simulink model "STATEFLOW"  (R2024b)
settings: Solver=FixedStepAuto  StartTime=0.0  StopTime=10.0  RelTol=1e-3  EnableMultiTasking=on
settings Model: DataDictionary=Master_Dictionary.sldd  EnableAccessToBaseWorkspace=off  Creator=torni  LastModifiedBy=Will
settings OptimizationCC: DefaultParameterBehavior=Inlined  EnhancedBackFolding=on  PassReuseOutputArgsAs=Individual arguments  ZeroExternalMemoryAtStartup=off  ZeroInternalMemoryAtStartup=off  MaxStackSize=8192  OptimizeBlockOrder=speed  DifferentSizesBufferReuse=on  OptimizationCustomize=off  EfficientTunableParamExpr=on
settings DebuggingCC: ParameterTunabilityLossMsg=error
settings HardwareCC: ProdBitPerPointer=32  ProdBitPerSizeT=32  ProdBitPerPtrDiffT=32  ProdLargestAtomicInteger=Long  ProdLargestAtomicFloat=Double  ProdWordSize=32  ProdLongLongMode=on  ProdHWDeviceType=ARM Compatible->ARM Cortex-M
settings SFSimCC: MATLABDynamicMemAlloc=off
settings RTWCC: Description=Embedded Coder  SystemTargetFile=ert.tlc  HardwareBoard=STM32H7xx Based (Single-core)  TemplateMakefile=ert_default_tmf  Toolchain=GNU Tools for ARM Embedded Processors
settings CodeAppCC: ForceParamTrailComments=on  IgnoreCustomStorageClasses=off  OperatorAnnotations=on  SimulinkDataObjDesc=on  SFDataObjDesc=on  InsertBlockDesc=on
settings ERTTargetCC: TargetLangStandard=C99 (ISO)  CodeReplacementLibrary=ARM Cortex-M  ExtModeTransport=3  ExtModeStaticAlloc=on  ExtModeStaticAllocSize=2048  ExtModeMexFile=ext_xcp  ExtModeIntrfLevel=Level2 - Open

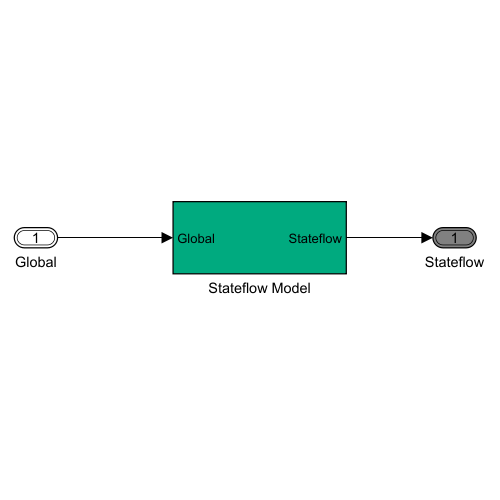
[thumbnail: Simulink's stored preview of the top-level diagram]
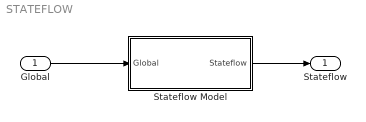
== system STATEFLOW ==
  "Global " : Inport  OutDataTypeStr=Bus: Global
  Stateflow Model : Subsystem
  Stateflow : Outport  OutDataTypeStr=Bus: Stateflow  VectorParamsAs1DForOutWhenUnconnected=off
  wires:
  "Global "/1 -> Stateflow Model/1(Global)
  Stateflow Model/1(Stateflow) -> Stateflow/1

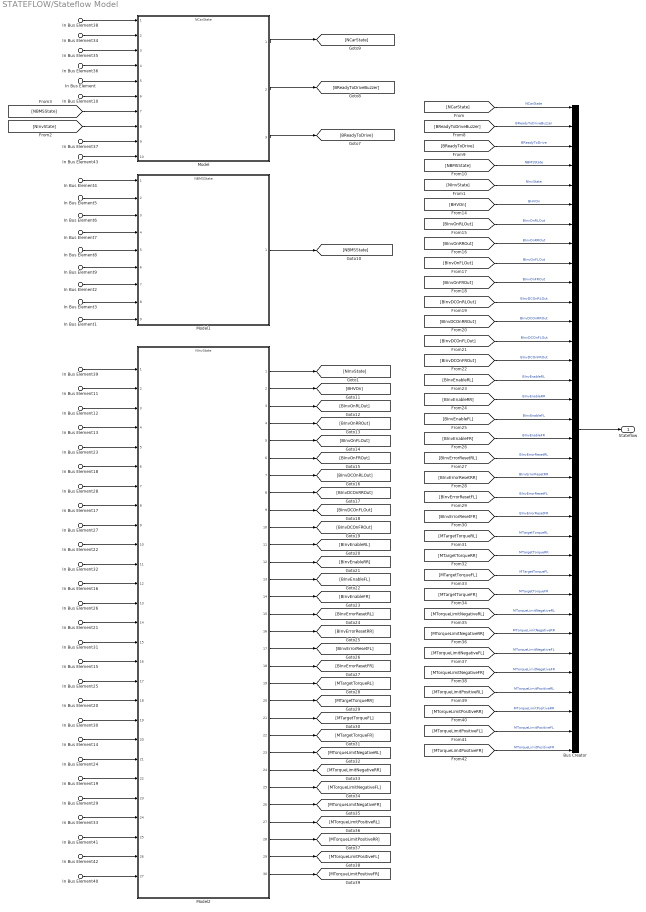
== system STATEFLOW/Stateflow Model ==
  In Bus Element : Inport  PortName=Global  Element=InverterSignals.InverterRLSignals.VDCInvRL
  In Bus Element11 : Inport  PortName=Global  Element=InverterSignals.InverterRLSignals.VDCInvRL
  In Bus Element10 : Inport  PortName=Global  Element=InverterSignals.InverterRLSignals.nMotorRL
  In Bus Element12 : Inport  PortName=Global  Element=InverterSignals.InverterRLSignals.nMotorRL
  In Bus Element13 : Inport  PortName=Global  Element=InverterSignals.InverterRLSignals.BInvErrorRL
  In Bus Element14 : Inport  PortName=Global  Element=InverterSignals.InverterRLSignals.BInvQuitDcOnRL
  In Bus Element15 : Inport  PortName=Global  Element=InverterSignals.InverterRLSignals.BQuitInvOnRL
  In Bus Element16 : Inport  PortName=Global  Element=InverterSignals.InverterRLSignals.BInvSysReadyRL
  In Bus Element17 : Inport  PortName=Global  Element=InverterSignals.InverterRLSignals.NInvDTCRL
  In Bus Element18 : Inport  PortName=Global  Element=InverterSignals.InverterFLSignals.BInvErrorFL
  In Bus Element19 : Inport  PortName=Global  Element=InverterSignals.InverterFLSignals.BInvQuitDcOnFL
  In Bus Element20 : Inport  PortName=Global  Element=InverterSignals.InverterFLSignals.BQuitInvOnFL
  In Bus Element21 : Inport  PortName=Global  Element=InverterSignals.InverterFLSignals.BInvSysReadyFL
  In Bus Element22 : Inport  PortName=Global  Element=InverterSignals.InverterFLSignals.NInvDTCFL
  In Bus Element40 : Inport  PortName=Global  Element=InverterSignals.InverterFLSignals.nMotorFL
  In Bus Element23 : Inport  PortName=Global  Element=InverterSignals.InverterRRSignals.BInvErrorRR
  In Bus Element24 : Inport  PortName=Global  Element=InverterSignals.InverterRRSignals.BInvQuitDcOnRR
  In Bus Element25 : Inport  PortName=Global  Element=InverterSignals.InverterRRSignals.BQuitInvOnRR
  In Bus Element26 : Inport  PortName=Global  Element=InverterSignals.InverterRRSignals.BInvSysReadyRR
  In Bus Element27 : Inport  PortName=Global  Element=InverterSignals.InverterRRSignals.NInvDTCRR
  In Bus Element41 : Inport  PortName=Global  Element=InverterSignals.InverterRRSignals.nMotorRR
  In Bus Element28 : Inport  PortName=Global  Element=InverterSignals.InverterFRSignals.BInvErrorFR
  In Bus Element29 : Inport  PortName=Global  Element=InverterSignals.InverterFRSignals.BInvQuitDcOnFR
  In Bus Element30 : Inport  PortName=Global  Element=InverterSignals.InverterFRSignals.BQuitInvOnFR
  In Bus Element31 : Inport  PortName=Global  Element=InverterSignals.InverterFRSignals.BInvSysReadyFR
  In Bus Element32 : Inport  PortName=Global  Element=InverterSignals.InverterFRSignals.NInvDTCFR
  In Bus Element42 : Inport  PortName=Global  Element=InverterSignals.InverterFRSignals.nMotorFR
  In Bus Element2 : Inport  PortName=Global  Element=BMSSignals.RCellAverage
  In Bus Element3 : Inport  PortName=Global  Element=BMSSignals.BBalancingOn
  In Bus Element4 : Inport  PortName=Global  Element=BMSSignals.BBMSP0A0C
  In Bus Element5 : Inport  PortName=Global  Element=BMSSignals.BBMSP0A0E
  In Bus Element6 : Inport  PortName=Global  Element=BMSSignals.BBMSP0A10
  In Bus Element7 : Inport  PortName=Global  Element=BMSSignals.BBMSP0A80
  In Bus Element8 : Inport  PortName=Global  Element=BMSSignals.BBMSP0AC0
  In Bus Element9 : Inport  PortName=Global  Element=BMSSignals.BBMSP0AFA
  In Bus Element33 : Inport  PortName=Global  Element=BMSSignals.VDCAccumulator
  In Bus Element1 : Inport  PortName=Global  Element=BMSSignals.VCellMin
  In Bus Element34 : Inport  PortName=Global  Element=Systems.rThrottlePedal
  In Bus Element35 : Inport  PortName=Global  Element=Systems.pBrakeF
  In Bus Element36 : Inport  PortName=Global  Element=Systems.pBrakeR
  In Bus Element37 : Inport  PortName=Global  Element=Systems.BReadyToDriveButton
  In Bus Element38 : Inport  PortName=Global  Element=Systems.BErrorReset
  In Bus Element39 : Inport  PortName=Global  Element=Systems.BErrorReset
  In Bus Element43 : Inport  PortName=Global  Element=Systems.BBrakeError
  Bus Creator : BusCreator  Inputs=34  OutDataTypeStr=Bus: Stateflow
  Model : ModelReference  ModelNameDialog=NCarState.slx  SimulationMode=Normal  ModelReferenceVersion=13.6
  Model1 : ModelReference  ModelNameDialog=NBMSState.slx  SimulationMode=Normal  ModelReferenceVersion=13.6
  Model2 : ModelReference  ModelNameDialog=NInvState.slx  SimulationMode=Normal  ModelReferenceVersion=13.6
  Stateflow : Outport  OutDataTypeStr=Bus: Stateflow  VectorParamsAs1DForOutWhenUnconnected=off
  wires:
  Model1/1 -> [NBMSState]
  In Bus Element4/1 -> Model1/1
  In Bus Element9/1 -> Model1/6
  In Bus Element7/1 -> Model1/4
  In Bus Element6/1 -> Model1/3
  In Bus Element5/1 -> Model1/2
  In Bus Element8/1 -> Model1/5
  Bus Creator/1 -> Stateflow/1
  In Bus Element2/1 -> Model1/7
  In Bus Element3/1 -> Model1/8
  In Bus Element34/1 -> Model/2
  In Bus Element35/1 -> Model/3
  In Bus Element36/1 -> Model/4
  In Bus Element/1 -> Model/5
  [NInvState] -> Model/8
  Model/1 -> [NCarState]
  Model/2 -> [BReadyToDriveBuzzer]
  Model/3 -> [BReadyToDrive]
  In Bus Element1/1 -> Model1/9
  In Bus Element39/1 -> Model2/1
  In Bus Element11/1 -> Model2/2
  In Bus Element12/1 -> Model2/3
  In Bus Element13/1 -> Model2/4
  In Bus Element23/1 -> Model2/5
  In Bus Element18/1 -> Model2/6
  In Bus Element28/1 -> Model2/7
  In Bus Element17/1 -> Model2/8
  In Bus Element27/1 -> Model2/9
  In Bus Element22/1 -> Model2/10
  In Bus Element32/1 -> Model2/11
  In Bus Element16/1 -> Model2/12
  In Bus Element26/1 -> Model2/13
  In Bus Element21/1 -> Model2/14
  In Bus Element31/1 -> Model2/15
  In Bus Element25/1 -> Model2/17
  In Bus Element20/1 -> Model2/18
  In Bus Element30/1 -> Model2/19
  In Bus Element15/1 -> Model2/16
  In Bus Element24/1 -> Model2/21
  In Bus Element19/1 -> Model2/22
  In Bus Element29/1 -> Model2/23
  Model2/1 -> [NInvState]
  Model2/2 -> [BHVOn]
  Model2/3 -> [BInvOnRLOut]
  Model2/4 -> [BInvOnRROut]
  Model2/5 -> [BInvOnFLOut]
  Model2/6 -> [BInvOnFROut]
  Model2/7 -> [BInvDCOnRLOut]
  Model2/8 -> [BInvDCOnRROut]
  Model2/9 -> [BInvDCOnFLOut]
  Model2/10 -> [BInvDCOnFROut]
  Model2/11 -> [BInvEnableRL]
  Model2/12 -> [BInvEnableRR]
  Model2/13 -> [BInvEnableFL]
  Model2/14 -> [BInvEnableFR]
  Model2/15 -> [BInvErrorResetRL]
  Model2/16 -> [BInvErrorResetRR]
  Model2/17 -> [BInvErrorResetFL]
  Model2/18 -> [BInvErrorResetFR]
  Model2/19 -> [MTargetTorqueRL]
  Model2/20 -> [MTargetTorqueRR]
  Model2/21 -> [MTargetTorqueFL]
  Model2/22 -> [MTargetTorqueFR]
  Model2/23 -> [MTorqueLimitNegativeRL]
  Model2/24 -> [MTorqueLimitNegativeRR]
  Model2/25 -> [MTorqueLimitNegativeFL]
  Model2/26 -> [MTorqueLimitNegativeFR]
  Model2/27 -> [MTorqueLimitPositiveRL]
  Model2/28 -> [MTorqueLimitPositiveRR]
  Model2/29 -> [MTorqueLimitPositiveFL]
  Model2/30 -> [MTorqueLimitPositiveFR]
  In Bus Element33/1 -> Model2/24
  In Bus Element10/1 -> Model/6
  In Bus Element14/1 -> Model2/20
  [NBMSState] -> Model/7
  In Bus Element38/1 -> Model/1
  In Bus Element37/1 -> Model/9
  [NBMSState] -> Bus Creator/4  "NBMSState"
  [BReadyToDriveBuzzer] -> Bus Creator/2  "BReadyToDriveBuzzer"
  [BReadyToDrive] -> Bus Creator/3  "BReadyToDrive"
  [NCarState] -> Bus Creator/1  "NCarState"
  [NInvState] -> Bus Creator/5  "NInvState"
  [BHVOn] -> Bus Creator/6  "BHVOn"
  [BInvOnRLOut] -> Bus Creator/7  "BInvOnRLOut"
  [BInvOnRROut] -> Bus Creator/8  "BInvOnRROut"
  [BInvOnFLOut] -> Bus Creator/9  "BInvOnFLOut"
  [BInvOnFROut] -> Bus Creator/10  "BInvOnFROut"
  [BInvDCOnRLOut] -> Bus Creator/11  "BInvDCOnRLOut"
  [BInvDCOnRROut] -> Bus Creator/12  "BInvDCOnRROut"
  [BInvDCOnFLOut] -> Bus Creator/13  "BInvDCOnFLOut"
  [BInvDCOnFROut] -> Bus Creator/14  "BInvDCOnFROut"
  [BInvEnableRL] -> Bus Creator/15  "BInvEnableRL"
  [BInvEnableRR] -> Bus Creator/16  "BInvEnableRR"
  [BInvEnableFL] -> Bus Creator/17  "BInvEnableFL"
  [BInvEnableFR] -> Bus Creator/18  "BInvEnableFR"
  [BInvErrorResetRL] -> Bus Creator/19  "BInvErrorResetRL"
  [BInvErrorResetRR] -> Bus Creator/20  "BInvErrorResetRR"
  [BInvErrorResetFL] -> Bus Creator/21  "BInvErrorResetFL"
  [BInvErrorResetFR] -> Bus Creator/22  "BInvErrorResetFR"
  [MTargetTorqueRL] -> Bus Creator/23  "MTargetTorqueRL"
  [MTargetTorqueRR] -> Bus Creator/24  "MTargetTorqueRR"
  [MTargetTorqueFL] -> Bus Creator/25  "MTargetTorqueFL"
  [MTargetTorqueFR] -> Bus Creator/26  "MTargetTorqueFR"
  [MTorqueLimitNegativeRL] -> Bus Creator/27  "MTorqueLimitNegativeRL"
  [MTorqueLimitNegativeRR] -> Bus Creator/28  "MTorqueLimitNegativeRR"
  [MTorqueLimitNegativeFL] -> Bus Creator/29  "MTorqueLimitNegativeFL"
  [MTorqueLimitNegativeFR] -> Bus Creator/30  "MTorqueLimitNegativeFR"
  [MTorqueLimitPositiveRL] -> Bus Creator/31  "MTorqueLimitPositiveRL"
  [MTorqueLimitPositiveRR] -> Bus Creator/32  "MTorqueLimitPositiveRR"
  [MTorqueLimitPositiveFL] -> Bus Creator/33  "MTorqueLimitPositiveFL"
  [MTorqueLimitPositiveFR] -> Bus Creator/34  "MTorqueLimitPositiveFR"
  In Bus Element40/1 -> Model2/27
  In Bus Element41/1 -> Model2/25
  In Bus Element42/1 -> Model2/26
  In Bus Element43/1 -> Model/10
